simulink model "valve_gas_test"  (R2017b)
settings: Solver=VariableStepAuto  StartTime=0.0  StopTime=0  RelTol=1e-3
undefined symbols (not defined in the file or in its folder): CoolProp
libraries: thermochemical x4
settings Model: Creator=ferru  LastModifiedBy=fferrucc

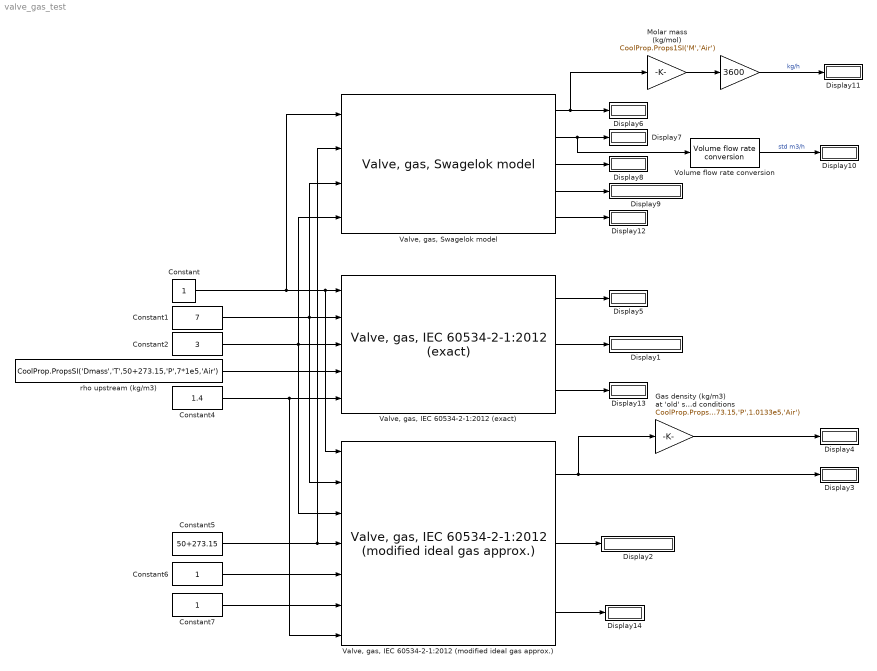
== system valve_gas_test ==
  " " : Gain  Gain=3600
  Constant : Constant
  Constant1 : Constant  Value=7
  Constant2 : Constant  Value=3
  Constant4 : Constant  Value=1.4
  Constant5 : Constant  Value=50+273.15
  Constant6 : Constant
  Constant7 : Constant
  Display{1..14} (14 alike) : Display
  Gas density (kg/m3) at 'old' standard conditions : Gain  Gain=CoolProp.PropsSI('Dmass','T',15.56+273.15,'P',1.0133e5,'Air')
  Molar mass (kg/mol) : Gain  Gain=CoolProp.Props1SI('M','Air')
  "Valve, gas, IEC 60534-2-1:2012 (exact)" : thermochemical/Valves/Valve, gas, IEC 60534-2-1:2012 (exact)  Cv_dataPoints=[0 0.01 0.02 0.05 0.09 0.1]  apperture_dataPoints=[0 0.2 0.4 0.6 0.8 1]  xT=0.5
      settings: SourceProductName=@ Thermochemical
  "Valve, gas, IEC 60534-2-1:2012 (modified ideal gas approx.)" : thermochemical/Valves/Valve, gas, IEC 60534-2-1:2012 (modified ideal gas approx.)  Cv_dataPoints=[0 0.01 0.02 0.05 0.09 0.1]  apperture_dataPoints=[0 0.2 0.4 0.6 0.8 1]  xT=0.5
      settings: SourceProductName=@ Thermochemical
  "Valve, gas, Swagelok model" : thermochemical/Valves/Valve, gas, Swagelok model  Cv_dataPoints=[0 0.01 0.02 0.05 0.09 0.1]  apperture_dataPoints=[0 0.2 0.4 0.6 0.8 1]  rho_gas_60F_1atm_kg_m3=CoolProp.PropsSI('Dmass','T',15.56+273.15,'P',1.0133e5,'Air')  M_gas=CoolProp.Props1SI('M','Air')
      settings: SourceProductName=@ Thermochemical
  Volume flow rate conversion : thermochemical/Conversions/Volume flow rate conversion  sel=CFH --> m3/h
      settings: SourceProductName=@ Thermochemical
  rho upstream (kg/m3) : Constant  Value=CoolProp.PropsSI('Dmass','T',50+273.15,'P',7*1e5,'Air')
  wires:
  Constant4/1 -> "Valve, gas, IEC 60534-2-1:2012 (modified ideal gas approx.)"/7, "Valve, gas, IEC 60534-2-1:2012 (exact)"/5
  rho upstream (kg/m3)/1 -> "Valve, gas, IEC 60534-2-1:2012 (exact)"/4
  Constant2/1 -> "Valve, gas, Swagelok model"/4, "Valve, gas, IEC 60534-2-1:2012 (modified ideal gas approx.)"/3, "Valve, gas, IEC 60534-2-1:2012 (exact)"/3
  Constant1/1 -> "Valve, gas, Swagelok model"/3, "Valve, gas, IEC 60534-2-1:2012 (modified ideal gas approx.)"/2, "Valve, gas, IEC 60534-2-1:2012 (exact)"/2
  "Valve, gas, IEC 60534-2-1:2012 (exact)"/1 -> Display5/1
  "Valve, gas, IEC 60534-2-1:2012 (exact)"/2 -> Display1/1
  Constant6/1 -> "Valve, gas, IEC 60534-2-1:2012 (modified ideal gas approx.)"/5
  Constant5/1 -> "Valve, gas, Swagelok model"/2, "Valve, gas, IEC 60534-2-1:2012 (modified ideal gas approx.)"/4
  "Valve, gas, IEC 60534-2-1:2012 (modified ideal gas approx.)"/1 -> Gas density (kg/m3) at 'old' standard conditions/1, Display3/1
  "Valve, gas, IEC 60534-2-1:2012 (modified ideal gas approx.)"/2 -> Display2/1
  Constant7/1 -> "Valve, gas, IEC 60534-2-1:2012 (modified ideal gas approx.)"/6
  Gas density (kg/m3) at 'old' standard conditions/1 -> Display4/1
  Constant/1 -> "Valve, gas, Swagelok model"/1, "Valve, gas, IEC 60534-2-1:2012 (modified ideal gas approx.)"/1, "Valve, gas, IEC 60534-2-1:2012 (exact)"/1
  "Valve, gas, Swagelok model"/3 -> Display8/1
  "Valve, gas, Swagelok model"/2 -> Volume flow rate conversion/1, Display7/1
  "Valve, gas, Swagelok model"/4 -> Display9/1
  Volume flow rate conversion/1 -> Display10/1  "std m3/h"
  Molar mass (kg/mol)/1 -> " "/1
  "Valve, gas, Swagelok model"/1 -> Molar mass (kg/mol)/1, Display6/1
  " "/1 -> Display11/1  "kg/h"
  "Valve, gas, Swagelok model"/5 -> Display12/1
  "Valve, gas, IEC 60534-2-1:2012 (exact)"/3 -> Display13/1
  "Valve, gas, IEC 60534-2-1:2012 (modified ideal gas approx.)"/3 -> Display14/1
